simulink library "BasicAudioLib"  (R2022b)
settings: Solver=VariableStepAuto  StartTime=0.0  StopTime=10.0  RelTol=1e-3
libraries: Tone x2, Balance x1, Mute x1, Volume x1
settings Model: Creator=ra1043664  LastModifiedBy=ra1043664
settings SolverCC: AlgebraicLoopSolver=TrustRegion
settings DataIOCC: ReturnWorkspaceOutputs=off
settings DebuggingCC: UnconnectedInputMsg=warning  UnconnectedOutputMsg=warning  UnconnectedLineMsg=warning  SFMachineParentedDataDiag=warning  ArithmeticOperatorsInVariantConditions=warning
settings ModelReferenceCC: EnableRefExpFcnMdlSchedulingChecks=on
settings SFSimCC: CustomCodeUndefinedFunction=UseInterfaceOnly

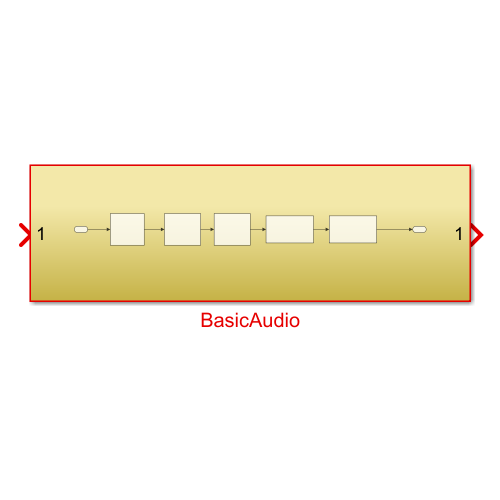
[thumbnail: Simulink's stored preview of the top-level diagram]
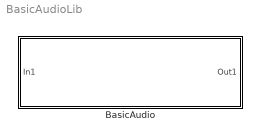
== system BasicAudioLib ==
  BasicAudio : Subsystem

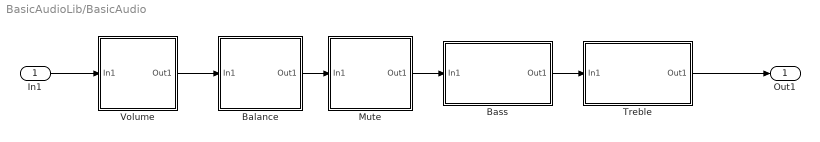
== system BasicAudioLib/BasicAudio ==
  In1 : Inport
  Balance : Subsystem  TreatAsAtomicUnit=on
  Bass : Subsystem  TreatAsAtomicUnit=on
  Mute : Subsystem  TreatAsAtomicUnit=on
  Treble : Subsystem  TreatAsAtomicUnit=on
  Volume : Subsystem  TreatAsAtomicUnit=on
  Out1 : Outport  VectorParamsAs1DForOutWhenUnconnected=off
  wires:
  In1/1 -> Volume/1(In1)
  Volume/1(Out1) -> Balance/1(In1)
  Balance/1(Out1) -> Mute/1(In1)
  Mute/1(Out1) -> Bass/1(In1)
  Bass/1(Out1) -> Treble/1(In1)
  Treble/1(Out1) -> Out1/1

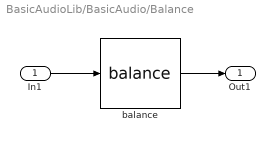
== system BasicAudioLib/BasicAudio/Balance ==
  In1 : Inport
  balance : Balance/balance  BankNumber=0  MaskFeatureName=Balance  MaskOffset=127  MaskChanRampMap="[1  2]"  MaskPackageNumber=2  MaskSilentExtreme=off  MaskSilentExtremeBass=on  MaskBoostDisable=off
  Out1 : Outport
  wires:
  balance/1 -> Out1/1
  In1/1 -> balance/1

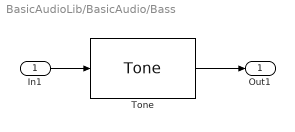
== system BasicAudioLib/BasicAudio/Bass ==
  In1 : Inport
  Tone : Tone/Tone  BankNumber=0  TriggerInit=[90 20 195 80]  MaskFeatureName=Bass  MaskFilterType=lowpass  MaskCutHz=200  MaskCut_dB=20  MaskBoostHz=200  MaskBoost_dB=20  MaskDefaultOffset=128  MaskDefaultScale=127  MaskPackageName=mode
  Out1 : Outport
  wires:
  Tone/1 -> Out1/1
  In1/1 -> Tone/1

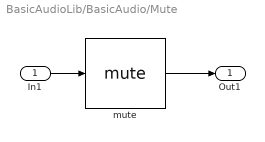
== system BasicAudioLib/BasicAudio/Mute ==
  In1 : Inport
  mute : Mute/mute  initial_mute_state=0  samplesPerFrame=32  MaskFeatureName=Mute
  Out1 : Outport
  wires:
  mute/1 -> Out1/1
  In1/1 -> mute/1

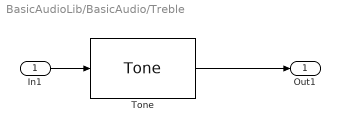
== system BasicAudioLib/BasicAudio/Treble ==
  In1 : Inport
  Tone : Tone/Tone  BankNumber=0  TriggerInit=[90 20 195 80]  MaskFeatureName=Treble  MaskFilterType=highpass  MaskCutHz=200  MaskCut_dB=20  MaskBoostHz=200  MaskBoost_dB=20  MaskDefaultOffset=128  MaskDefaultScale=127  MaskPackageName=mode
  Out1 : Outport
  wires:
  In1/1 -> Tone/1
  Tone/1 -> Out1/1

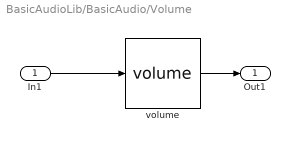
== system BasicAudioLib/BasicAudio/Volume ==
  In1 : Inport
  volume : Volume/volume  initial_linear_gain=0  LastName=Volume  PackageName=mode  BankNumber=0  TriggerInit=[120 20 195 90]  MaskFeatureName=Volume  MaskEnableGainOutput=off  MaskRows=8  MaskVolumeTable=[0 -100; 0.5 -30; 1 0]
  Out1 : Outport
  wires:
  volume/1 -> Out1/1
  In1/1 -> volume/1
